simulink model "multi_susp_sys_comps"  (Simulink 7.7)
settings: Solver=ode45  StartTime=0.0  StopTime=5000  RelTol=1e-3
undefined symbols (not defined in the file): G, s, Suspension, suspension_lib
libraries: simulink x3
settings Model: Creator=jporter  LastModifiedBy=jporter

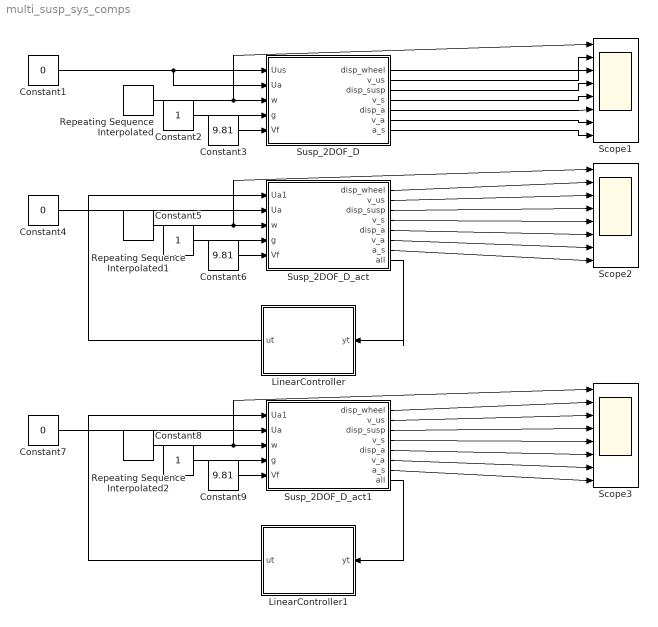
== system multi_susp_sys_comps ==
  Constant1 : Constant  Value=0
  Constant2 : Constant
  Constant3 : Constant  Value=9.81
  Constant4 : Constant  Value=0
  Constant5 : Constant
  Constant6 : Constant  Value=9.81
  Constant7 : Constant  Value=0
  Constant8 : Constant
  Constant9 : Constant  Value=9.81
  LinearController : Subsystem
  LinearController1 : Subsystem
  Repeating Sequence Interpolated : simulink/Sources/Repeating Sequence Interpolated  SystemSampleTime=-1  OutValues=[0 0.5 0 -0.5 0 -0.5 0 0.5 0].'  TimeValues=[0 0.1 0.2 0.3 0.4 0.6 0.7 0.8 0.9].'  LookUpMeth=Interpolation-Use End Values  tsamp=0.01  OutMin=[]  OutMax=[]  OutDataTypeStr=double  OutputDataTypeScalingMode=double  OutDataType=fixdt(0,8)  OutScaling=2^-10
  Repeating Sequence Interpolated1 : simulink/Sources/Repeating Sequence Interpolated  SystemSampleTime=-1  OutValues=[0 0.5 0 -0.5 0 -0.5 0 0.5 0].'  TimeValues=[0 0.1 0.2 0.3 0.4 0.6 0.7 0.8 0.9].'  LookUpMeth=Interpolation-Use End Values  tsamp=0.01  OutMin=[]  OutMax=[]  OutDataTypeStr=double  OutputDataTypeScalingMode=double  OutDataType=fixdt(0,8)  OutScaling=2^-10
  Repeating Sequence Interpolated2 : simulink/Sources/Repeating Sequence Interpolated  SystemSampleTime=-1  OutValues=[0 0.5 0 -0.5 0 -0.5 0 0.5 0].'  TimeValues=[0 0.1 0.2 0.3 0.4 0.6 0.7 0.8 0.9].'  LookUpMeth=Interpolation-Use End Values  tsamp=0.01  OutMin=[]  OutMax=[]  OutDataTypeStr=double  OutputDataTypeScalingMode=double  OutDataType=fixdt(0,8)  OutScaling=2^-10
  Scope1 : Scope  NumInputPorts=8
      settings: YMin=-0.5~-0.5~-30~-0.9~-5~-5~-5~-5  YMax=0.5~0.5~30~0.3~5~5~5~5
  Scope2 : Scope  NumInputPorts=8
      settings: YMin=-0.5~-0.5~-30~-0.9~-5~-5~-5~-5  YMax=0.5~0.5~30~0.3~5~5~5~5
  Scope3 : Scope  NumInputPorts=8
      settings: YMin=-0.5~-0.5~-30~-0.9~-5~-5~-5~-5  YMax=0.5~0.5~30~0.3~5~5~5~5  SaveName=ScopeData2
  Susp_2DOF_D : Subsystem  AncestorBlock=suspension_lib/Suspension:G(s)  mask{m_s=25000, k_s=60000, b_s=3500, m_us=413, k_us=65096.03, b_us=15000, m_a=0, k_a=0, b_a=0}
      mask prompts: m_s "Sprung mass (kg)"; k_s "Sprung mass spring constant (N/m)"; b_s "Sprung mass damping coefficient (N s/m)"; m_us "Unsprung mass (kg)"; k_us "Unsprung mass spring constant (N/m)"; b_us "Unsprung mass damping coefficient (N s/m)"; m_a "Damper mass (kg)"; k_a "Damper spring constant (N/m)"; b_a "Damper damping coeff (N s/m)"
      mask init:
      | w = sqrt( k_us / m_us );
      | w_us = sqrt( k_us / m_us );
      | rho = m_s / m_us;
      | rho_a = 0;
      | g = 9.81; % m/s^2 gravitational acceleration
      | 
      | % m_s == 0 and m_us == 0 are not allowed
      | % Work around possible divide by zero when m_a == 0
      | %  build A by rows
      | A = [0 1 0 0 0 0]; 
      | A = [A; -(k_us/m_us) (-b_s/m_us)+(b_us/m_us) (k_s/m_us) (b_s/m_us) 0 0]; 
      | A = [A; 0 -1 0 1 0 0]; 
      | A = [A; 0 (b_s/m_s) -(k_s/m_s) (-b_s/m_s) 0 0];
      | if ( m_a ~= 0 )
      |   w_a = sqrt( k_a / m_a );
      |   eta_a = b_a / (2 * m_a * w_a);
      |   rho_a = m_us / m_a;  
      |   A = [A; 0 -1 0 0 0 1]; 
      |   A = [A; 0 2 * eta_a * w_a 0 0 -(w_a^2) -2 * eta_a * w_a];
      | else
      |   A = [A; 0 0 0 0 0 0];
      |   A = [A; 0 0 0 0 0 0];
      | end
      | 
      | A=-A;
      | 
      | % inputs: active damper control force, 
      | %   active suspension control force,
      | %   road velocity, gravity, and sprung mass force
      | B = [0 0 -1 0 0];
      | B = [B; rho rho -(b_us/m_us) -g 0];
      | B = [B; 0 0 0 0 0];
      | B = [B; 0 -1 0 0 -1];
      | B = [B; 0 0 0 0 0];
      | B = [B; -rho * rho_a 0 0 0 0];
      | 
      | 
      | % A = [0 1 0 0 0 0]; 
      | % A = [A; -(k_us/m_us)  (-b_a/m_us) 0 0 (k_a/m_us) (b_a/m_us)]; 
      | % A = [A; 0 -1 0 1 0 0]; 
      | % A = [A; 0 0 0 0 0 0];
      | % if ( m_a ~= 0 )
      | %   w_a = sqrt( k_a / m_a );
      | %   eta_a = b_a / (2 * m_a * w_a);
      | %   rho_a = m_us / m_a;  
      | %   A = [A; 0 -1 0 0 0 1]; 
      | %   A = [A; 0 2 * eta_a * w_a 0 0 -(w_a^2) -2 * eta_a * w_a];
      | % else
      | %   A = [A; 0 0 0 0 0 0];
      | %   A = [A; 0 0 0 0 0 0];
      | % end
  Susp_2DOF_D_act : Subsystem  AncestorBlock=suspension_lib/Suspension:G(s)  mask{m_s=25000, k_s=60000, b_s=3500, m_us=413, k_us=65096.03, b_us=15000, m_a=0, k_a=0, b_a=0}
      mask prompts: m_s "Sprung mass (kg)"; k_s "Sprung mass spring constant (N/m)"; b_s "Sprung mass damping coefficient (N s/m)"; m_us "Unsprung mass (kg)"; k_us "Unsprung mass spring constant (N/m)"; b_us "Unsprung mass damping coefficient (N s/m)"; m_a "Damper mass (kg)"; k_a "Damper spring constant (N/m)"; b_a "Damper damping coeff (N s/m)"
      mask init: same as multi_susp_sys_comps/Susp_2DOF_D
  Susp_2DOF_D_act1 : Subsystem  AncestorBlock=suspension_lib/Suspension:G(s)  mask{m_s=25000, k_s=60000, b_s=3500, m_us=413, k_us=65096.03, b_us=15000, m_a=0, k_a=0, b_a=0}
      mask prompts: m_s "Sprung mass (kg)"; k_s "Sprung mass spring constant (N/m)"; b_s "Sprung mass damping coefficient (N s/m)"; m_us "Unsprung mass (kg)"; k_us "Unsprung mass spring constant (N/m)"; b_us "Unsprung mass damping coefficient (N s/m)"; m_a "Damper mass (kg)"; k_a "Damper spring constant (N/m)"; b_a "Damper damping coeff (N s/m)"
      mask init: same as multi_susp_sys_comps/Susp_2DOF_D
  wires:
  Repeating Sequence Interpolated/1 -> Susp_2DOF_D/3(w), Scope1/1
  Susp_2DOF_D/1(disp_wheel) -> Scope1/2
  Susp_2DOF_D/2(v_us) -> Scope1/3
  Susp_2DOF_D/3(disp_susp) -> Scope1/4
  Susp_2DOF_D/4(v_s) -> Scope1/5
  Susp_2DOF_D/5(disp_a) -> Scope1/6
  Susp_2DOF_D/6(v_a) -> Scope1/7
  Constant1/1 -> Susp_2DOF_D/1(Uus), Susp_2DOF_D/2(Ua)
  Constant2/1 -> Susp_2DOF_D/4(g)
  Constant3/1 -> Susp_2DOF_D/5(Vf)
  Susp_2DOF_D/7(a_s) -> Scope1/8
  Repeating Sequence Interpolated1/1 -> Susp_2DOF_D_act/3(w), Scope2/1
  Susp_2DOF_D_act/1(disp_wheel) -> Scope2/2
  Susp_2DOF_D_act/2(v_us) -> Scope2/3
  Susp_2DOF_D_act/3(disp_susp) -> Scope2/4
  Susp_2DOF_D_act/4(v_s) -> Scope2/5
  Susp_2DOF_D_act/5(disp_a) -> Scope2/6
  Susp_2DOF_D_act/6(v_a) -> Scope2/7
  Constant4/1 -> Susp_2DOF_D_act/2(Ua)
  Constant5/1 -> Susp_2DOF_D_act/4(g)
  Constant6/1 -> Susp_2DOF_D_act/5(Vf)
  Susp_2DOF_D_act/7(a_s) -> Scope2/8
  Susp_2DOF_D_act/8(all) -> LinearController/1(yt)
  LinearController/1(ut) -> Susp_2DOF_D_act/1(Ua1)
  Repeating Sequence Interpolated2/1 -> Susp_2DOF_D_act1/3(w), Scope3/1
  Susp_2DOF_D_act1/1(disp_wheel) -> Scope3/2
  Susp_2DOF_D_act1/2(v_us) -> Scope3/3
  Susp_2DOF_D_act1/3(disp_susp) -> Scope3/4
  Susp_2DOF_D_act1/4(v_s) -> Scope3/5
  Susp_2DOF_D_act1/5(disp_a) -> Scope3/6
  Susp_2DOF_D_act1/6(v_a) -> Scope3/7
  Constant7/1 -> Susp_2DOF_D_act1/2(Ua)
  Constant8/1 -> Susp_2DOF_D_act1/4(g)
  Constant9/1 -> Susp_2DOF_D_act1/5(Vf)
  Susp_2DOF_D_act1/7(a_s) -> Scope3/8
  Susp_2DOF_D_act1/8(all) -> LinearController1/1(yt)
  LinearController1/1(ut) -> Susp_2DOF_D_act1/1(Ua1)

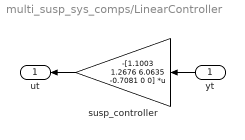
== system multi_susp_sys_comps/LinearController ==
  yt : Inport
  susp_controller : Gain  Gain=-[1.1003 1.2676 6.0635 -0.7081 0 0]  Multiplication=Matrix(K*u)
  ut : Outport
  wires:
  yt/1 -> susp_controller/1
  susp_controller/1 -> ut/1

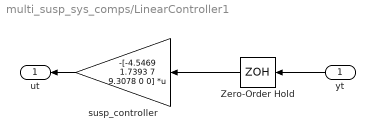
== system multi_susp_sys_comps/LinearController1 ==
  yt : Inport
  Zero-Order Hold : ZeroOrderHold  SampleTime=0.01
  susp_controller : Gain  Gain=-[-4.5469 1.7393 7 9.3078 0 0]  Multiplication=Matrix(K*u)
  ut : Outport
  wires:
  yt/1 -> Zero-Order Hold/1
  susp_controller/1 -> ut/1
  Zero-Order Hold/1 -> susp_controller/1

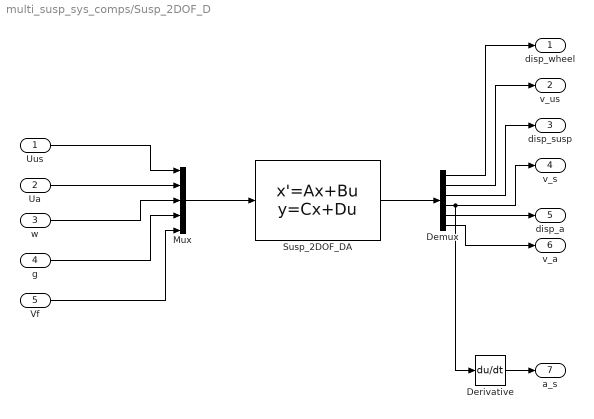
== system multi_susp_sys_comps/Susp_2DOF_D ==
  Uus : Inport
  Ua : Inport  Port=2
  w : Inport  Port=3
  g : Inport  Port=4
  Vf : Inport  Port=5
  Demux : Demux  Outputs=6
  Derivative : Derivative
  Mux : Mux  Inputs=5
  Susp_2DOF_DA : StateSpace  A=A  B=B  C=eye(6)  D=zeros(6,5)
  disp_wheel : Outport
  v_us : Outport  Port=2
  disp_susp : Outport  Port=3
  v_s : Outport  Port=4
  disp_a : Outport  Port=5
  v_a : Outport  Port=6
  a_s : Outport  Port=7
  wires:
  Uus/1 -> Mux/1
  Ua/1 -> Mux/2
  w/1 -> Mux/3
  Mux/1 -> Susp_2DOF_DA/1
  Susp_2DOF_DA/1 -> Demux/1
  Demux/1 -> disp_wheel/1
  Demux/2 -> v_us/1
  Demux/3 -> disp_susp/1
  Demux/4 -> v_s/1, Derivative/1
  Demux/5 -> disp_a/1
  Demux/6 -> v_a/1
  g/1 -> Mux/4
  Vf/1 -> Mux/5
  Derivative/1 -> a_s/1

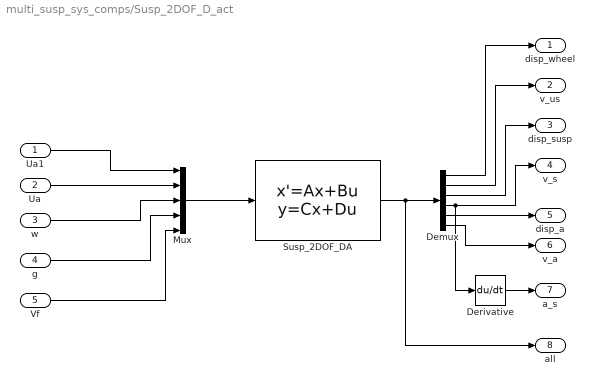
== system multi_susp_sys_comps/Susp_2DOF_D_act ==
  Ua1 : Inport
  Ua : Inport  Port=2
  w : Inport  Port=3
  g : Inport  Port=4
  Vf : Inport  Port=5
  Demux : Demux  Outputs=6
  Derivative : Derivative
  Mux : Mux  Inputs=5
  Susp_2DOF_DA : StateSpace  A=A  B=B  C=eye(6)  D=zeros(6,5)
  disp_wheel : Outport
  v_us : Outport  Port=2
  disp_susp : Outport  Port=3
  v_s : Outport  Port=4
  disp_a : Outport  Port=5
  v_a : Outport  Port=6
  a_s : Outport  Port=7
  all : Outport  Port=8
  wires:
  Ua/1 -> Mux/2
  w/1 -> Mux/3
  Mux/1 -> Susp_2DOF_DA/1
  Susp_2DOF_DA/1 -> Demux/1, all/1
  Demux/1 -> disp_wheel/1
  Demux/2 -> v_us/1
  Demux/3 -> disp_susp/1
  Demux/4 -> v_s/1, Derivative/1
  Demux/5 -> disp_a/1
  Demux/6 -> v_a/1
  g/1 -> Mux/4
  Vf/1 -> Mux/5
  Derivative/1 -> a_s/1
  Ua1/1 -> Mux/1

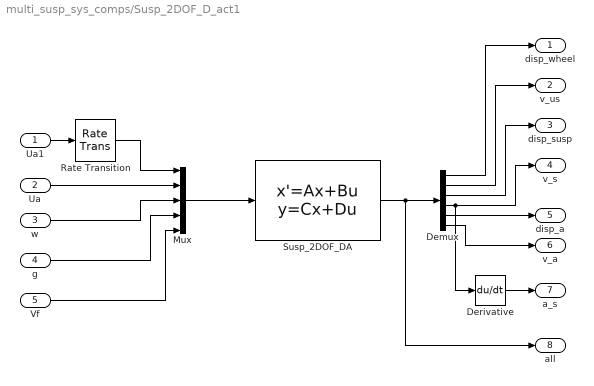
== system multi_susp_sys_comps/Susp_2DOF_D_act1 ==
  Ua1 : Inport
  Ua : Inport  Port=2
  w : Inport  Port=3
  g : Inport  Port=4
  Vf : Inport  Port=5
  Demux : Demux  Outputs=6
  Derivative : Derivative
  Mux : Mux  Inputs=5
  Rate Transition : RateTransition
  Susp_2DOF_DA : StateSpace  A=A  B=B  C=eye(6)  D=zeros(6,5)
  disp_wheel : Outport
  v_us : Outport  Port=2
  disp_susp : Outport  Port=3
  v_s : Outport  Port=4
  disp_a : Outport  Port=5
  v_a : Outport  Port=6
  a_s : Outport  Port=7
  all : Outport  Port=8
  wires:
  Ua/1 -> Mux/2
  w/1 -> Mux/3
  Mux/1 -> Susp_2DOF_DA/1
  Susp_2DOF_DA/1 -> Demux/1, all/1
  Demux/1 -> disp_wheel/1
  Demux/2 -> v_us/1
  Demux/3 -> disp_susp/1
  Demux/4 -> v_s/1, Derivative/1
  Demux/5 -> disp_a/1
  Demux/6 -> v_a/1
  g/1 -> Mux/4
  Vf/1 -> Mux/5
  Derivative/1 -> a_s/1
  Ua1/1 -> Rate Transition/1
  Rate Transition/1 -> Mux/1
